simulink model "PMSMSMO"  (R2014b)
settings: Solver=ode45  StartTime=0.0  StopTime=1  RelTol=1e-3
InitFcn:
  | run Parameters;
undefined symbols (not defined in the file or in its folder): i_limit, J, Ld, Lq, np, psi_f, Rs, Ts, Ts_ACR, Ts_ASR, u_limit
undefined symbols (not defined in the file): ki_ACRd, ki_ACRq, kp_ACRd, kp_ACRq, kz_ASR
libraries: powerlib x11, simulink x1
settings Model: Creator=Zhaoxuqiang  LastModifiedBy=Zhaoxuqiang

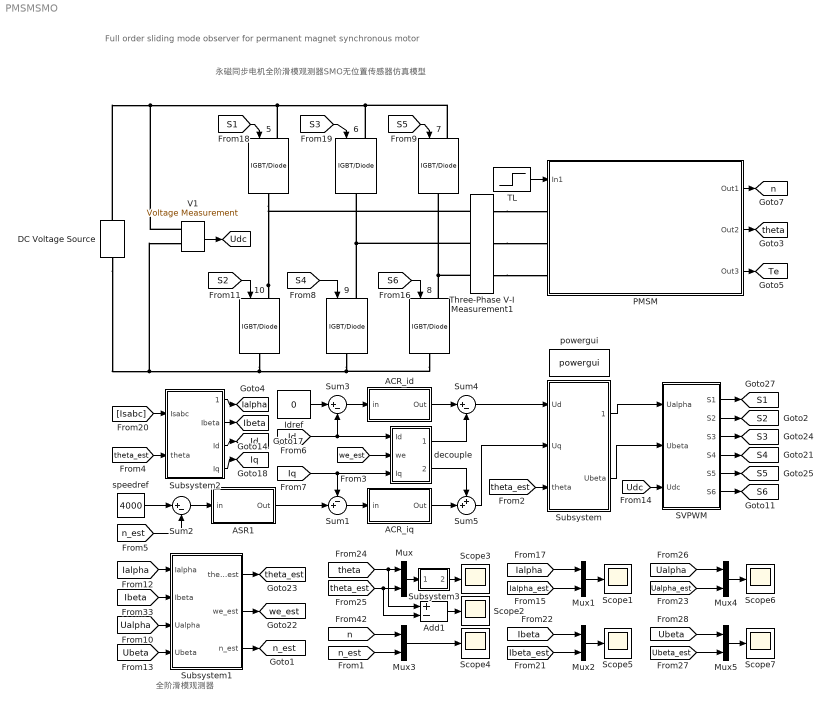
== system PMSMSMO ==
  note: 全阶滑模观测器
  note: Full order sliding mode observer for permanent magnet synchronous motor
  note: 永磁同步电机全阶滑模观测器SMO无位置传感器仿真模型
  {5..10} (6 alike) : powerlib/Power Electronics/IGBT//Diode  Ron=1e-3  Rs=5000  Cs=inf  Measurements=off
  ACR_id : Subsystem  mask{kp=kp_ACRd, ki=ki_ACRd, Ts=Ts_ACR}
      mask Display: disp('PI');
  ACR_iq : Subsystem  mask{kp=kp_ACRq, ki=ki_ACRq, Ts=Ts_ACR}
      mask Display: disp('PI');
  ASR1 : Subsystem  mask{kp=0.01, ki=1.5, kz=kz_ASR, i_limit=i_limit, Ts=Ts_ASR}
      mask Display: disp('PI');
  Add1 : Sum  Inputs=+-
  DC Voltage Source : powerlib/Electrical Sources/DC Voltage Source  Amplitude=310  Measurements=None
  Idref : Constant  Value=0  SampleTime=Ts_ASR
  Mux{,1..5} (6 alike) : Mux  Inputs=2
  PMSM : Subsystem
      mask Display: image('PMSM.jpg');
  SVPWM : Subsystem  mask{fs=1e4}
  Scope{1..7} (7 alike) : Scope
      Scope1 settings: YMin=0  YMax=10000  SaveName=ScopeData5
      Scope2 settings: YMin=-1  YMax=1
      Scope3 settings: YMin=-1  YMax=8  SaveName=ScopeData8
      Scope4 settings: YMin=0  YMax=4000  SaveName=ScopeData3
      Scope5 settings: YMin=0  YMax=10000  SaveName=ScopeData6
      Scope6 settings: YMin=0  YMax=10000  SaveName=ScopeData7
      Scope7 settings: YMin=0  YMax=10000  SaveName=ScopeData9
  Subsystem : Subsystem
  Subsystem1 : Subsystem
  Subsystem2 : Subsystem
  Subsystem3 : Subsystem
  Sum1 : Sum  Inputs=-+|
  Sum2 : Sum  Inputs=|+-
  Sum3 : Sum  Inputs=|+-
  Sum4 : Sum  Inputs=|+-
  Sum5 : Sum  Inputs=++|
  TL : Step  Time=0.15  SampleTime=0
  Three-Phase V-I Measurement1 : powerlib/Measurements/Three-Phase V-I Measurement  VoltageMeasurement=phase-to-phase  SetLabelV=on  LabelV=Usabc  Vpu=off  VpuLL=off  CurrentMeasurement=yes  SetLabelI=on  LabelI=Isabc  Ipu=off  Pbase=100e6  Vbase=500e3  OutputType=Complex  PhasorSimulation=off  PSBequivalent=0
  V1 : powerlib/Measurements/Voltage Measurement  PhasorSimulation=off  OutputType=Complex  PSBequivalent=0
  decouple : Subsystem  mask{psi_f=psi_f, Ld=Ld, Lq=Lq}
  powergui : powerlib/powergui  Priority=1  SimulationMode=Discrete  SolverType=Backward Euler  SampleTime=Ts  frequency=60  SPID=off  DisableSnubberDevices=off  DisableRonSwitches=off  DisableVfSwitches=off  SwTol=0  DisplayEquations=off  Interpol=off  methode=off  Ts=0  frequencyindice=0  Pbase=100e6  ErrMax=1e-4  Iterations=50  UnitsV=kV  UnitsW=MW  FunctionMessages=off  echomessages=off  HookPort=off  EnableUseOfTLC=off  x0status=blocks  RestoreLinks=warning  ResistiveCurrentMeasurement=off  Frange=[0:2:500]  Ylog=off  Xlog=on  ShowGrid=off  save=off  variable=ZData  structure=Iin  ZoomFFT=on  StartTime=0.4  cycles=4  DisplayStyle=1  fundamental=50  FreqAxis=on  MaxFrequency=1050  frequencyindicesteady=1  RmsSteady=1  display=off
  speedref : Constant  Value=4000  SampleTime=Ts_ASR
  tag scope: Ialpha=global, Ibeta=global, Id=global, Iq=global, S1=global, S2=global, S3=global, S4=global, S5=global, S6=global, Te=global, Udc=global, n=global, n_est=global, theta=global, theta_est=global, we_est=global
  wires:
  V1/1 -> [Udc]
  [Udc] -> SVPWM/3(Udc)
  Sum1/1 -> ACR_iq/1(in)
  Idref/1 -> Sum3/1
  Sum2/1 -> ASR1/1(in)
  [Id] -> Sum3/2, decouple/1(Id)
  Sum3/1 -> ACR_id/1(in)
  speedref/1 -> Sum2/1
  ACR_id/1(Out) -> Sum4/1
  ACR_iq/1(Out) -> Sum5/2
  ASR1/1(Out) -> Sum1/2
  [Iq] -> Sum1/1, decouple/3(Iq)
  [we_est] -> decouple/2(we)
  decouple/1(ud1) -> Sum4/2
  decouple/2(uq2) -> Sum5/1
  Sum4/1 -> Subsystem/1(Ud)
  Sum5/1 -> Subsystem/2(Uq)
  [theta_est] -> Subsystem/3(theta)
  Subsystem/1(Ualpha) -> SVPWM/1(Ualpha)
  Subsystem/2(Ubeta) -> SVPWM/2(Ubeta)
  [n_est] -> Sum2/2
  [Ialpha] -> Subsystem1/1(Ialpha)
  [Ibeta] -> Subsystem1/2(Ibeta)
  [Ualpha] -> Subsystem1/3(Ualpha)
  [Ubeta] -> Subsystem1/4(Ubeta)
  Subsystem1/1(theta_est) -> [theta_est]
  Subsystem1/2(we_est) -> [we_est]
  Subsystem1/3(n_est) -> [n_est]
  [S1] -> 5/1
  [S2] -> 10/1
  [S3] -> 6/1
  [S4] -> 9/1
  [S5] -> 7/1
  [S6] -> 8/1
  SVPWM/1(S1) -> [S1]
  SVPWM/2(S2) -> [S2]
  SVPWM/3(S3) -> [S3]
  SVPWM/4(S4) -> [S4]
  SVPWM/5(S5) -> [S5]
  SVPWM/6(S6) -> [S6]
  [Isabc] -> Subsystem2/1(Isabc)
  [theta_est] -> Subsystem2/2(theta)
  Subsystem2/1(Ialpha) -> [Ialpha]
  Subsystem2/2(Ibeta) -> [Ibeta]
  Subsystem2/3(Id) -> [Id]
  Subsystem2/4(Iq) -> [Iq]
  [n] -> Mux3/1
  [n_est] -> Mux3/2
  Mux3/1 -> Scope4/1
  [theta] -> Add1/1, Mux/1
  [theta_est] -> Add1/2, Mux/2
  Mux/1 -> Subsystem3/1(1)
  Subsystem3/1(2) -> Scope3/1
  Add1/1 -> Scope2/1
  [Ialpha_est] -> Mux1/2
  Mux1/1 -> Scope1/1
  [Ialpha] -> Mux1/1
  [Ibeta_est] -> Mux2/2
  Mux2/1 -> Scope5/1
  [Ibeta] -> Mux2/1
  [Ualpha_est] -> Mux4/2
  Mux4/1 -> Scope6/1
  [Ualpha] -> Mux4/1
  [Ubeta_est] -> Mux5/2
  Mux5/1 -> Scope7/1
  [Ubeta] -> Mux5/1
  TL/1 -> PMSM/1(In1)
  PMSM/1(Out1) -> [n]
  PMSM/2(Out2) -> [theta]
  PMSM/3(Out3) -> [Te]
  connections:
  Three-Phase V-I Measurement1/LConn2 -- 9/LConn1 -- 6/RConn1
  10/LConn1 -- 5/RConn1 -- Three-Phase V-I Measurement1/LConn1
  Three-Phase V-I Measurement1/LConn3 -- 8/LConn1 -- 7/RConn1
  DC Voltage Source/LConn1 -- V1/LConn2 -- 10/RConn1 -- 8/RConn1 -- 9/RConn1
  DC Voltage Source/RConn1 -- V1/LConn1 -- 5/LConn1 -- 7/LConn1 -- 6/LConn1
  Three-Phase V-I Measurement1/RConn1 -- PMSM/LConn1
  Three-Phase V-I Measurement1/RConn2 -- PMSM/LConn2
  Three-Phase V-I Measurement1/RConn3 -- PMSM/LConn3

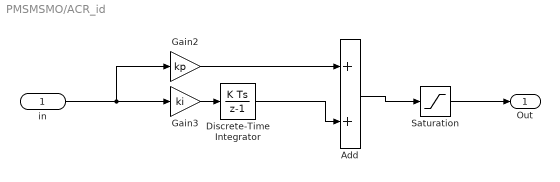
== system PMSMSMO/ACR_id ==
  in : Inport
  Add : Sum
  Discrete-Time Integrator : DiscreteIntegrator  SampleTime=Ts
  Gain2 : Gain  Gain=kp
  Gain3 : Gain  Gain=ki
  Saturation : Saturate  UpperLimit=u_limit  LowerLimit=-u_limit  SampleTime=Ts
  Out : Outport
  wires:
  in/1 -> Gain2/1, Gain3/1
  Gain2/1 -> Add/1
  Gain3/1 -> Discrete-Time Integrator/1
  Add/1 -> Saturation/1
  Discrete-Time Integrator/1 -> Add/2
  Saturation/1 -> Out/1

== system PMSMSMO/ACR_iq ==
  in : Inport
  Add : Sum
  Discrete-Time Integrator : DiscreteIntegrator  SampleTime=Ts
  Gain2 : Gain  Gain=kp
  Gain3 : Gain  Gain=ki
  Saturation : Saturate  UpperLimit=u_limit  LowerLimit=-u_limit  SampleTime=Ts
  Out : Outport
  wires:
  in/1 -> Gain2/1, Gain3/1
  Gain2/1 -> Add/1
  Gain3/1 -> Discrete-Time Integrator/1
  Add/1 -> Saturation/1
  Discrete-Time Integrator/1 -> Add/2
  Saturation/1 -> Out/1

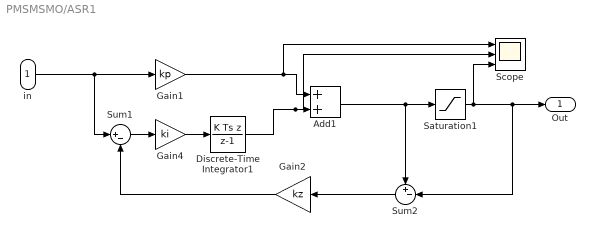
== system PMSMSMO/ASR1 ==
  in : Inport
  Add1 : Sum
  Discrete-Time Integrator1 : DiscreteIntegrator  IntegratorMethod=Integration: Backward Euler  SampleTime=Ts  UpperSaturationLimit=3  LowerSaturationLimit=-3
  Gain1 : Gain  Gain=kp  SampleTime=Ts
  Gain2 : Gain  Gain=kz  SampleTime=Ts
  Gain4 : Gain  Gain=ki  SampleTime=Ts
  Saturation1 : Saturate  UpperLimit=i_limit  LowerLimit=-i_limit  SampleTime=Ts
  Scope : Scope  NumInputPorts=3
  Sum1 : Sum  Inputs=|+-
  Sum2 : Sum  Inputs=+-|
  Out : Outport
  wires:
  Gain1/1 -> Scope/1, Add1/1
  Add1/1 -> Saturation1/1, Sum2/1
  in/1 -> Sum1/1, Gain1/1
  Saturation1/1 -> Scope/3, Sum2/2, Out/1
  Sum2/1 -> Gain2/1
  Discrete-Time Integrator1/1 -> Scope/2, Add1/2
  Gain4/1 -> Discrete-Time Integrator1/1
  Sum1/1 -> Gain4/1
  Gain2/1 -> Sum1/2

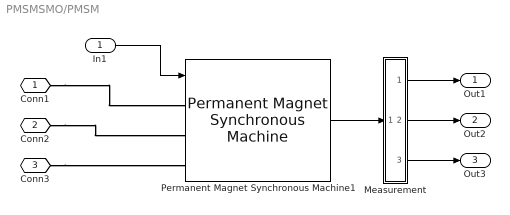
== system PMSMSMO/PMSM ==
  In1 : Inport
  Measurement : Subsystem
  Permanent Magnet Synchronous Machine1 : powerlib/Machines/Permanent Magnet Synchronous Machine  NbPhases=3  FluxDistribution=Sinusoidal  RotorType=Salient-pole  MechanicalLoad=Torque Tm  PresetModel=No  ShowDetailedParameters=on  MeasurementBus=off  Resistance=Rs  Inductance=8.5e-3  dqInductances=[Ld,Lq]  La=Lq  MachineConstant=Flux linkage established by magnets (V.s)  Flux=psi_f  VoltageCst=36.276  TorqueCst=0.3  Flat=120  Mechanical=[J 0 np 0.3]  PolePairs=np  InitialConditions=[0,0, 0,0]  InitialConditions5ph=[0 0 0 0 0 0]  TsPowergui=0  TsBlock=Ts  RefAngle=Aligned with phase A axis (original Park)
  Conn1 : PMIOPort  Port=1  Side=Left
  Conn2 : PMIOPort  Port=2  Side=Left
  Conn3 : PMIOPort  Port=3  Side=Left
  Out1 : Outport
  Out2 : Outport  Port=2
  Out3 : Outport  Port=3
  wires:
  Measurement/2(theta) -> Out2/1
  Measurement/3(Te) -> Out3/1
  Permanent Magnet Synchronous Machine1/1 -> Measurement/1(M)
  In1/1 -> Permanent Magnet Synchronous Machine1/1
  Measurement/1(n) -> Out1/1
  connections:
  Conn2/RConn1 -- Permanent Magnet Synchronous Machine1/LConn2
  Conn3/RConn1 -- Permanent Magnet Synchronous Machine1/LConn3
  Conn1/RConn1 -- Permanent Magnet Synchronous Machine1/LConn1

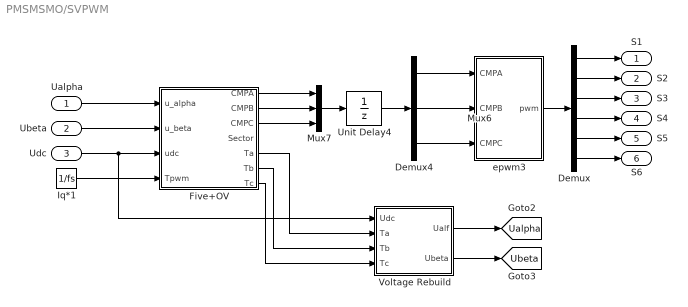
== system PMSMSMO/SVPWM ==
  Ualpha : Inport
  Ubeta : Inport  Port=2
  Udc : Inport  Port=3
  Demux : Demux  Outputs=6
  Demux4 : Demux  Outputs=3
  Five+OV : MATLAB Function  TreatAsAtomicUnit=on
  Iq*1 : Constant  Value=1/fs
  Mux6 : Mux  Inputs=3
  Mux7 : Mux  Inputs=3
  Unit Delay4 : UnitDelay  SampleTime=Ts_ACR
  Voltage Rebuild : MATLAB Function  TreatAsAtomicUnit=on
  epwm3 : Subsystem
  S1 : Outport
  S2 : Outport  Port=2
  S3 : Outport  Port=3
  S4 : Outport  Port=4
  S5 : Outport  Port=5
  S6 : Outport  Port=6
  tag scope: Ualpha=global, Ubeta=global
  wires:
  Demux4/2 -> epwm3/2(CMPB)
  Demux4/3 -> epwm3/3(CMPC)
  Five+OV/1(CMPA) -> Mux7/1
  Five+OV/2(CMPB) -> Mux7/2
  Five+OV/3(CMPC) -> Mux7/3
  Mux7/1 -> Unit Delay4/1
  Unit Delay4/1 -> Demux4/1
  Demux4/1 -> epwm3/1(CMPA)
  Iq*1/1 -> Five+OV/4(Tpwm)
  Udc/1 -> Voltage Rebuild/1(Udc), Five+OV/3(udc)
  Ubeta/1 -> Five+OV/2(u_beta)
  Ualpha/1 -> Five+OV/1(u_alpha)
  Five+OV/5(Ta) -> Voltage Rebuild/2(Ta)
  Five+OV/6(Tb) -> Voltage Rebuild/3(Tb)
  Five+OV/7(Tc) -> Voltage Rebuild/4(Tc)
  Voltage Rebuild/1(Ualf) -> [Ualpha]
  Voltage Rebuild/2(Ubeta) -> [Ubeta]
  epwm3/1(pwm) -> Demux/1
  Demux/1 -> S1/1
  Demux/2 -> S2/1
  Demux/3 -> S3/1
  Demux/4 -> S4/1
  Demux/5 -> S5/1
  Demux/6 -> S6/1

== system PMSMSMO/Subsystem ==
  Ud : Inport
  Uq : Inport  Port=2
  theta : Inport  Port=3
  ipark : MATLAB Function  TreatAsAtomicUnit=on
  Ualpha : Outport
  Ubeta : Outport  Port=2
  wires:
  Ud/1 -> ipark/1(ud)
  ipark/1(u_alpha) -> Ualpha/1
  ipark/2(u_beta) -> Ubeta/1
  theta/1 -> ipark/3(theta)
  Uq/1 -> ipark/2(uq)

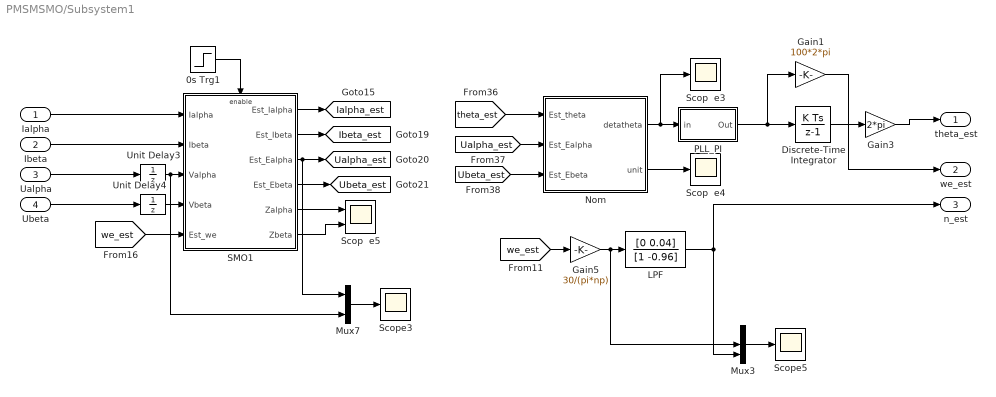
== system PMSMSMO/Subsystem1 ==
  Ialpha : Inport
  Ibeta : Inport  Port=2
  Ualpha : Inport  Port=3
  Ubeta : Inport  Port=4
  0s Trg1 : Step  Time=0.0001  SampleTime=0
  Discrete-Time Integrator : DiscreteIntegrator  gainval=100  SampleTime=-1
  Gain1 : Gain  Gain=100*2*pi
  Gain3 : Gain  Gain=2*pi
  Gain5 : Gain  Gain=30/(pi*np)
  LPF : DiscreteFilter  Numerator=[0 0.04]  Denominator=[1 -0.96]  SampleTime=1e-4
  Mux3 : Mux  Inputs=3
  Mux7 : Mux  Inputs=2
  Nom : MATLAB Function  TreatAsAtomicUnit=on
  PLL_PI : Subsystem  mask{kp=1, ki=50, Ts=Ts_ACR}
  SMO1 : Subsystem  mask{Rs=Rs, Ld=Ld, Lq=Lq, k=18, m=180, Ts=Ts_ACR, Tpu=Ts_ACR, tao=1}
  Scop  e3 : Scope
  Scop  e4 : Scope
  Scop  e5 : Scope  NumInputPorts=2
      settings: YMin=-5~-5  YMax=5~5
  Scope3 : Scope
      settings: YMin=-100  YMax=100  SaveName=ScopeData2
  Scope5 : Scope
      settings: YMin=500  YMax=5000  SaveName=ScopeData4
  Unit Delay3 : UnitDelay  SampleTime=Ts_ACR
  Unit Delay4 : UnitDelay  SampleTime=Ts_ACR
  theta_est : Outport
  we_est : Outport  Port=2
  n_est : Outport  Port=3
  tag scope: Ialpha_est=global, Ibeta_est=global, Ualpha_est=global, Ubeta_est=global
  wires:
  Mux7/1 -> Scope3/1
  Ialpha/1 -> SMO1/1(Ialpha)
  Ibeta/1 -> SMO1/2(Ibeta)
  Unit Delay3/1 -> Mux7/2, SMO1/3(Valpha)
  Unit Delay4/1 -> SMO1/4(Vbeta)
  0s Trg1/1 -> SMO1/Enable
  Ualpha/1 -> Unit Delay3/1
  Ubeta/1 -> Unit Delay4/1
  SMO1/1(Est_Ialpha) -> [Ialpha_est]
  SMO1/2(Est_Ibeta) -> [Ibeta_est]
  SMO1/3(Est_Ealpha) -> Mux7/1, [Ualpha_est]
  SMO1/4(Est_Ebeta) -> [Ubeta_est]
  SMO1/5(Zalpha) -> Scop  e5/1
  SMO1/6(Zbeta) -> Scop  e5/2
  Discrete-Time Integrator/1 -> Gain3/1
  [theta_est] -> Nom/1(Est_theta)
  [Ualpha_est] -> Nom/2(Est_Ealpha)
  [Ubeta_est] -> Nom/3(Est_Ebeta)
  Nom/1(detatheta) -> PLL_PI/1(in), Scop  e3/1
  Nom/2(unit) -> Scop  e4/1
  Gain3/1 -> theta_est/1
  PLL_PI/1(Out) -> Discrete-Time Integrator/1, Gain1/1
  Gain1/1 -> we_est/1
  [we_est] -> SMO1/5(Est_we)
  Mux3/1 -> Scope5/1
  [we_est] -> Gain5/1
  LPF/1 -> n_est/1, Mux3/3
  ? -> Mux3/1
  Gain5/1 -> Mux3/2, LPF/1

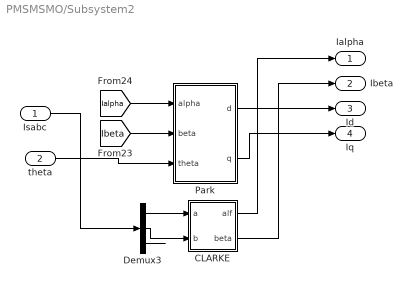
== system PMSMSMO/Subsystem2 ==
  Isabc : Inport
  theta : Inport  Port=2
  CLARKE : MATLAB Function  TreatAsAtomicUnit=on
  Demux3 : Demux  Outputs=3
  Park : MATLAB Function  TreatAsAtomicUnit=on
  Ialpha : Outport
  Ibeta : Outport  Port=2
  Id : Outport  Port=3
  Iq : Outport  Port=4
  wires:
  Demux3/2 -> CLARKE/2(b)
  Isabc/1 -> Demux3/1
  CLARKE/1(alf) -> Ialpha/1
  CLARKE/2(beta) -> Ibeta/1
  Demux3/1 -> CLARKE/1(a)
  [Ibeta] -> Park/2(beta)
  [Ialpha] -> Park/1(alpha)
  Park/2(q) -> Iq/1
  Park/1(d) -> Id/1
  theta/1 -> Park/3(theta)
  Demux3/3 -> ?

== system PMSMSMO/Subsystem3 ==
  1 : Inport
  2*pi : Constant  Value=2*pi  SampleTime=Ts_ASR
  Math Function2 : Math  Operator=mod  RndMeth=Zero  SaturateOnIntegerOverflow=on
  2 : Outport
  wires:
  Math Function2/1 -> 2/1
  2*pi/1 -> Math Function2/2
  1/1 -> Math Function2/1

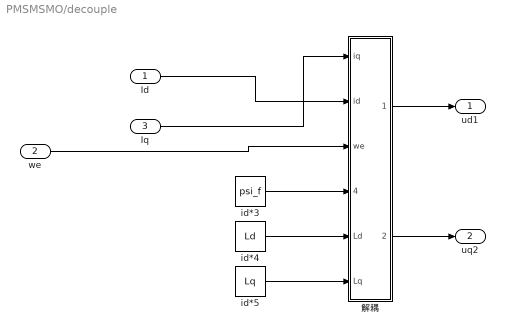
== system PMSMSMO/decouple ==
  Id : Inport
  we : Inport  Port=2
  Iq : Inport  Port=3
  id*3 : Constant  Value=psi_f
  id*4 : Constant  Value=Ld
  id*5 : Constant  Value=Lq
  解耦 : MATLAB Function  TreatAsAtomicUnit=on
  ud1 : Outport
  uq2 : Outport  Port=2
  wires:
  we/1 -> 解耦/3(we)
  id*5/1 -> 解耦/6(Lq)
  id*4/1 -> 解耦/5(Ld)
  id*3/1 -> 解耦/4(psi_f)
  解耦/2(uq_c) -> uq2/1
  Iq/1 -> 解耦/1(iq)
  Id/1 -> 解耦/2(id)
  解耦/1(ud_c) -> ud1/1

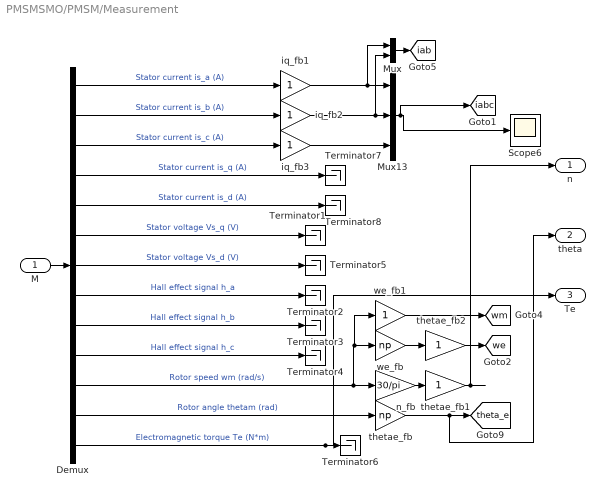
== system PMSMSMO/PMSM/Measurement ==
  M : Inport
  Demux : Demux  Outputs=13
  Mux : Mux  Inputs=2
  Mux13 : Mux  Inputs=3
  Scope6 : Scope
      settings: YMin=0  YMax=10000  SaveName=ScopeData10
  Terminator{1..8} (8 alike) : Terminator
  iq_fb1 : Gain  SampleTime=Ts_ACR
  iq_fb2 : Gain  SampleTime=Ts_ACR
  iq_fb3 : Gain  SampleTime=Ts_ACR
  n_fb : Gain  Gain=30/pi  SampleTime=Ts_ASR
  thetae_fb : Gain  Gain=np  SampleTime=Ts_ACR
  thetae_fb1 : Gain  SampleTime=Ts_ASR
  thetae_fb2 : Gain  SampleTime=Ts_ASR
  we_fb : Gain  Gain=np  SampleTime=Ts_ASR
  we_fb1 : Gain  SampleTime=Ts_ASR
  n : Outport
  theta : Outport  Port=2
  Te : Outport  Port=3
  tag scope: iab=global, iabc=global, theta_e=global, we=global, wm=global
  wires:
  thetae_fb2/1 -> [we]
  thetae_fb1/1 -> n/1
  Mux13/1 -> [iabc], Scope6/1
  iq_fb3/1 -> Mux13/3
  Demux/3 -> iq_fb3/1  "Stator current is_c (A)"
  Demux/2 -> iq_fb2/1  "Stator current is_b (A)"
  Demux/1 -> iq_fb1/1  "Stator current is_a (A)"
  iq_fb1/1 -> Mux/1, Mux13/1
  we_fb1/1 -> [wm]
  we_fb/1 -> thetae_fb2/1
  Demux/7 -> Terminator5/1  "Stator voltage Vs_d (V)"
  Demux/6 -> Terminator1/1  "Stator voltage Vs_q (V)"
  n_fb/1 -> thetae_fb1/1
  thetae_fb/1 -> theta/1, [theta_e]
  Demux/5 -> Terminator8/1  "Stator current is_d (A)"
  Demux/4 -> Terminator7/1  "Stator current is_q (A)"
  Demux/9 -> Terminator3/1  "Hall effect signal h_b"
  Demux/13 -> Te/1, Terminator6/1  "Electromagnetic torque Te (N*m)"
  Demux/8 -> Terminator2/1  "Hall effect signal h_a"
  Demux/11 -> n_fb/1, we_fb/1, we_fb1/1  "Rotor speed wm (rad/s)"
  Demux/12 -> thetae_fb/1  "Rotor angle thetam (rad)"
  Demux/10 -> Terminator4/1  "Hall effect signal h_c"
  M/1 -> Demux/1
  iq_fb2/1 -> Mux/2, Mux13/2
  Mux/1 -> [iab]

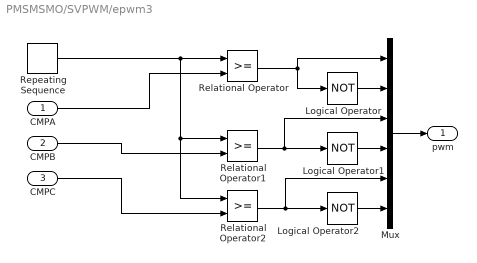
== system PMSMSMO/SVPWM/epwm3 ==
  CMPA : Inport
  CMPB : Inport  Port=2
  CMPC : Inport  Port=3
  Logical Operator : Logic  Operator=NOT  AllPortsSameDT=off  OutDataTypeStr=boolean
  Logical Operator1 : Logic  Operator=NOT  AllPortsSameDT=off  OutDataTypeStr=boolean
  Logical Operator2 : Logic  Operator=NOT  AllPortsSameDT=off  OutDataTypeStr=boolean
  Mux : Mux  Inputs=6
  Relational Operator : RelationalOperator  OutDataTypeStr=boolean
  Relational Operator1 : RelationalOperator  OutDataTypeStr=boolean
  Relational Operator2 : RelationalOperator  OutDataTypeStr=boolean
  Repeating Sequence : simulink/Sources/Repeating Sequence  rep_seq_t=[0 1/fs/2 1/fs]  rep_seq_y=[0 1/(2*fs) 0]
  pwm : Outport
  wires:
  Repeating Sequence/1 -> Relational Operator/1, Relational Operator2/1, Relational Operator1/1
  Relational Operator1/1 -> Logical Operator1/1, Mux/3
  Logical Operator/1 -> Mux/2
  Mux/1 -> pwm/1
  Logical Operator1/1 -> Mux/4
  Logical Operator2/1 -> Mux/6
  CMPA/1 -> Relational Operator/2
  CMPB/1 -> Relational Operator1/2
  CMPC/1 -> Relational Operator2/2
  Relational Operator/1 -> Logical Operator/1, Mux/1
  Relational Operator2/1 -> Logical Operator2/1, Mux/5

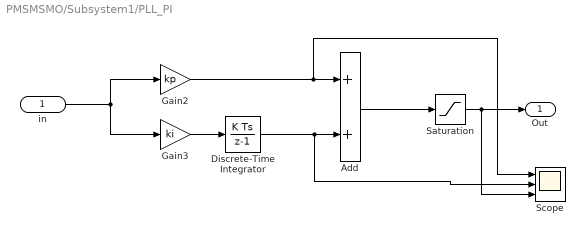
== system PMSMSMO/Subsystem1/PLL_PI ==
  in : Inport
  Add : Sum
  Discrete-Time Integrator : DiscreteIntegrator  SampleTime=Ts
  Gain2 : Gain  Gain=kp
  Gain3 : Gain  Gain=ki
  Saturation : Saturate  UpperLimit=inf  LowerLimit=-inf
  Scope : Scope  NumInputPorts=3
  Out : Outport
  wires:
  Gain2/1 -> Scope/1, Add/1
  Gain3/1 -> Discrete-Time Integrator/1
  Discrete-Time Integrator/1 -> Scope/2, Add/2
  in/1 -> Gain3/1, Gain2/1
  Add/1 -> Saturation/1
  Saturation/1 -> Scope/3, Out/1

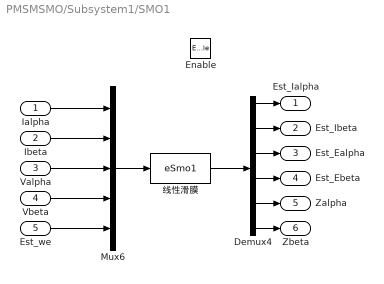
== system PMSMSMO/Subsystem1/SMO1 ==
  Ialpha : Inport
  Ibeta : Inport  Port=2
  Valpha : Inport  Port=3
  Vbeta : Inport  Port=4
  Est_we : Inport  Port=5
  Enable : EnablePort
  Demux4 : Demux  Outputs=6
  Mux6 : Mux  Inputs=5
  线性滑膜 : S-Function  FunctionName=eSmo1  Parameters=Rs,Ld,Lq,k,m,Ts,Tpu,tao  EnableBusSupport=off
  Est_Ialpha : Outport
  Est_Ibeta : Outport  Port=2
  Est_Ealpha : Outport  Port=3
  Est_Ebeta : Outport  Port=4
  Zalpha : Outport  Port=5
  Zbeta : Outport  Port=6
  wires:
  Vbeta/1 -> Mux6/4
  Valpha/1 -> Mux6/3
  Ialpha/1 -> Mux6/1
  Ibeta/1 -> Mux6/2
  Demux4/4 -> Est_Ebeta/1
  Demux4/1 -> Est_Ialpha/1
  Demux4/3 -> Est_Ealpha/1
  Demux4/2 -> Est_Ibeta/1
  Est_we/1 -> Mux6/5
  线性滑膜/1 -> Demux4/1
  Mux6/1 -> 线性滑膜/1
  Demux4/5 -> Zalpha/1
  Demux4/6 -> Zbeta/1

== matlab function PMSMSMO/Subsystem1/Nom ==
  data: detatheta output; Est_theta input; Est_Ealpha input; Est_Ebeta input; unit output
function [detatheta,unit]  = fcn(Est_theta,Est_Ealpha,Est_Ebeta)
%#codegen
deta=-cos(Est_theta)*Est_Ealpha-sin(Est_theta)*Est_Ebeta;

unit=sqrt(Est_Ealpha*Est_Ealpha+Est_Ebeta*Est_Ebeta);
%归一化
if(unit<5)
    unit=5;
end

detatheta=deta/unit;

== matlab function PMSMSMO/Subsystem/ipark ==
  data: u_alpha output; ud input; uq input; u_beta output; theta input
function [u_alpha,u_beta] = fcn(ud,uq,theta)
%#codegen
u_alpha=ud*cos(theta)-uq*sin(theta);
u_beta=ud*sin(theta)+uq*cos(theta);

== matlab function PMSMSMO/decouple/解耦 ==
  data: iq input; ud_c output; uq_c output; id input; we input; psi_f input; Ld input; Lq input
function [ud_c,uq_c] = fcn(iq,id,we,psi_f,Ld,Lq)

%#codegen
uq_c=we*(Ld*id+psi_f);
ud_c=we*Lq*iq;

== matlab function PMSMSMO/Subsystem2/CLARKE ==
  data: a input; alf output; b input; beta output
function [alf,beta] = clarke(a,b)
alf = a;
beta = (2*b+a)/(sqrt(3));

== matlab function PMSMSMO/SVPWM/Five+OV ==
  data: CMPA output; u_alpha input; u_beta input; udc input; Tpwm input; CMPB output; CMPC output; Sector output; Ta output; Tb output; Tc output
function [CMPA,CMPB,CMPC,Sector,Ta,Tb,Tc] = fcn(u_alpha,u_beta,udc,Tpwm)
%#Copyright HUST 
CMPA=0;
CMPB=0;
CMPC=0;
Ta=0;
Tb=0;
Tc=0;

sqrt32=(sqrt(3))/2;
sqrt3=sqrt(3);
m=sqrt3/udc;

X=u_beta;
Y=(sqrt32*u_alpha+0.5*u_beta);
Z=Y-X;

    Sector=3;
    if Y>0
        Sector=Sector-1;
    end
    if Z>0
        Sector=Sector-1;
    end
    if X<0
        Sector=7-Sector;
    end		
  
    if(Sector==1)
         Ta=m*Y;														
         Tb=m*X; 												
         Tc=0;
         temp=Ta;
    if(temp>=1)
         Ta=Ta/temp;
         Tb=Tb/temp;
    end
        CMPA=(1-Ta)*(Tpwm/2);
        CMPB=(1-Tb)*(Tpwm/2);
        CMPC=(1-Tc)*(Tpwm/2);
    end		

    if( Sector==2)
         Ta=m*Y;														
         Tb=m*X; 												
         Tc=0;
         temp=Tb;
    if(temp>=1)
         Ta=Ta/temp;
         Tb=Tb/temp;
    end		
        CMPA=(1-Ta)*(Tpwm/2);
        CMPB=(1-Tb)*(Tpwm/2);
        CMPC=(1-Tc)*(Tpwm/2);
    end	
   																				
    if(Sector==3)                                  
        Ta= 0; 												
        Tb= m*(-Z); 														
      	Tc= m*(-Y);
        temp=Tb;
    if(temp>=1)
         Tb=Tb/temp;
         Tc=Tc/temp;
    end
        CMPA=(1-Ta)*(Tpwm/2);
        CMPB=(1-Tb)*(Tpwm/2);
        CMPC=(1-Tc)*(Tpwm/2);
    end

    if(Sector==4)                                  
        Ta= 0; 												
        Tb= m*(-Z); 														
      	Tc= m*(-Y);
         temp=Tc;
    if(temp>=1)
         Tb=Tb/temp;
         Tc=Tc/temp;
    end
        CMPA=(1-Ta)*(Tpwm/2);
        CMPB=(1-Tb)*(Tpwm/2);
        CMPC=(1-Tc)*(Tpwm/2);
    end
    
    if(Sector==5)
           Ta= m*Z; 														
      	   Tb= 0; 														
      	   Tc= m*(-X);
         temp=Tc;
    if(temp>=1)
         Ta=Ta/temp;
         Tc=Tc/temp;
    end
        CMPA=(1-Ta)*(Tpwm/2);
        CMPB=(1-Tb)*(Tpwm/2);
        CMPC=(1-Tc)*(Tpwm/2);
    end

    if(Sector==6)
           Ta= m*Z; 														
      	   Tb= 0; 														
      	   Tc= m*(-X);
         temp=Ta;
    if(temp>=1)
         Ta=Ta/temp;
         Tc=Tc/temp;
    end
        CMPA=(1-Ta)*(Tpwm/2);
        CMPB=(1-Tb)*(Tpwm/2);
        CMPC=(1-Tc)*(Tpwm/2);
    end

== matlab function PMSMSMO/Subsystem2/Park ==
  data: d output; alpha input; beta input; q output; theta input
function [d,q] = fcn(alpha,beta,theta)
%#codegen
d=alpha*cos(theta)+beta*sin(theta);
q=-alpha*sin(theta)+beta*cos(theta);

== matlab function PMSMSMO/SVPWM/Voltage Rebuild ==
  data: Udc input; Ualf output; Ta input; Ubeta output; Tb input; Tc input
function [Ualf,Ubeta] = f(Udc,Ta,Tb,Tc)

temp=Udc/3;
va=(2*Ta-Tb-Tc)*temp;
vb=(2*Tb-Ta-Tc)*temp;
Ualf=va;
Ubeta=(va+2*vb)/sqrt(3);
